simulink model "SMC_seg_tray_forma2"  (R2026b)
settings: Solver=ode4  StopTime=20  FixedStep=0.0001
settings Model: Creator=nestorhernandezcastellanos  LastModifiedBy=nestorhernandezcastellanos

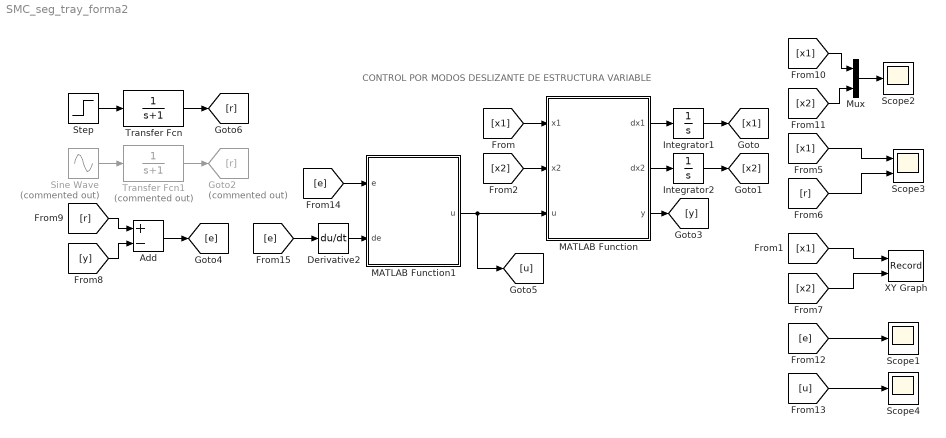
== system SMC_seg_tray_forma2 ==
  note: CONTROL POR MODOS DESLIZANTE DE ESTRUCTURA VARIABLE
  Add : Sum  Inputs=+-
  Derivative2 : Derivative
  Goto2 : Goto  Commented=on  GotoTag=r
  Integrator1 : Integrator  InitialCondition=1
  Integrator2 : Integrator  InitialCondition=-2
  MATLAB Function : MATLAB Function  TreatAsAtomicUnit=on
  MATLAB Function1 : MATLAB Function  TreatAsAtomicUnit=on
  Mux : Mux  Inputs=2
  Scope1 : Scope
      settings: ActiveDisplayYMinimum=-1.1345018827917306  ActiveDisplayYMaximum=0.21051694512557476
  Scope2 : Scope
      settings: ActiveDisplayYMinimum=-2.3780113002128531  ActiveDisplayYMaximum=1.4021017019156774  DataLoggingVariableName=ScopeData2
  Scope3 : Scope  NumInputPorts=2
      settings: ActiveDisplayYMinimum=-0.12500113839065802  ActiveDisplayYMaximum=1.1250102455159223  DataLoggingVariableName=ScopeData3
  Scope4 : Scope
      settings: ActiveDisplayYMinimum=-16.499792391312006  ActiveDisplayYMaximum=12.498131521808045
  Sine Wave : Sin  Commented=on  SampleTime=0
  Step : Step  Time=10  SampleTime=0
  Transfer Fcn : TransferFcn  Denominator=[1 1]
  Transfer Fcn1 : TransferFcn  Commented=on  Denominator=[1 1]
  XY Graph : Record  NumPorts=2.0  FileSettingsInternal="{\"entries\":[{\"content\":{\"excelSettings\":{\"content\":{},\"type\":\"Streamout.ExcelSettings\"},\"parquetSettings\":{\"content\":{},\"type\":\"Streamout.ParquetSettings\"}},\"type\":\"Streamout.FileSettingStorage\",\"uuid\":\"\"}],\"packageUris\":[\"http:\\/\\/schema.mathworks.com\\/mf0\\/streamout_blocks\\/R2020a\"],\"version\":\"1.0\"}"  FrameSettings=[0, 0]  Layout=[1 1]  SignalsInternal="{\"entries\":[{\"content\":{\"signals\":[{\"content\":{\"blockPath\":[],\"dimensions\":[1],\"domain\":\"\",\"lineColor\":\"#a2142f\",\"plots\":[ 1 ],\"port\":1,\"signalID\":1,\"signalName\":\"From1\"},\"type\":\"RecordBlkView.Signal\",\"uuid\":\"\"},{\"content\":{\"blockPath\":[],\"dimensions\":[1],\"domain\":\"\",\"lineColor\":\"#139fff\",\"plots\":[ 1 ],\"port\":2,\"signalID\":2,\"signalName\":\"From7\"},\"type\":\"RecordBlkView.Signal\",\"uuid\":\"\"}]},\"type\":\"RecordBlkView.InputSignals\",\"uuid\":\"\"}],\"packageUris\":[\"http:\\/\\/schema.mathworks.com\\/mf0\\/streamout_blocks\\/R2020a\"],\"version\":\"1.0\"}"  VisualizationBindings="{\"xyplotplugin\":{\"info\":[{\"series\":[{\"bindingParametersList\":[{\"parameter\":\"X-Axis\",\"signalID\":1,\"signalName\":\"From1\"},{\"parameter\":\"Y-Axis\",\"signalID\":2,\"signalName\":\"From7\"}],\"seriesID\":0}],\"subplotID\":1}]}}"  CompatibilityTag=XY
  wires:
  MATLAB Function1/1(u) -> [u], MATLAB Function/3(u)
  MATLAB Function/2(dx2) -> Integrator2/1
  MATLAB Function/1(dx1) -> Integrator1/1
  Mux/1 -> Scope2/1
  Sine Wave/1 -> Transfer Fcn1/1
  Derivative2/1 -> MATLAB Function1/2(de)
  [x1] -> MATLAB Function/1(x1)
  [x1] -> XY Graph/1
  [x2] -> MATLAB Function/2(x2)
  [x1] -> Scope3/1
  [r] -> Scope3/2
  [x2] -> XY Graph/2
  Integrator2/1 -> [x2]
  Integrator1/1 -> [x1]
  MATLAB Function/3(y) -> [y]
  [y] -> Add/2
  [r] -> Add/1
  [x2] -> Mux/2
  [x1] -> Mux/1
  [e] -> Scope1/1
  [u] -> Scope4/1
  Add/1 -> [e]
  [e] -> MATLAB Function1/1(e)
  [e] -> Derivative2/1
  Step/1 -> Transfer Fcn/1
  Transfer Fcn/1 -> [r]
  Transfer Fcn1/1 -> Goto2/1

== matlab function SMC_seg_tray_forma2/MATLAB Function1 ==
  data: e input; de input; u output
function u = controlador(e, de)

% Ganancia K>1
K = 3;

% Valor arbitrario positivo
m = 2;
L = 0.8; % Amplitud máxima de mi sistema

s = de + m*e;
u = m*s + K*abs(L+m*m*e)*sign(s);

== matlab function SMC_seg_tray_forma2/MATLAB Function ==
  data: x1 input; x2 input; dx1 output; u input; dx2 output; y output
function [dx1, dx2, y] = planta(x1, x2, u)

dx1 = x2;
dx2 = sin(x1+x2) + cos(x1*x2) + u;

y = x1;
